simulink model "bldcm_model"  (R2023b)
settings: Solver=ode23s  StartTime=0.0  StopTime=10  RelTol=1e-3
libraries: spsMosfetLib x6, eeGeneralControl x3, simulink x1, spsDCVoltageSourceLib x1, spsGroundLib x1, slpidlib x1, spsThreePhaseSeriesRLCBranchLib x1, spsThreePhaseVIMeasurementLib x1, sps_lib x1
settings Model: Creator=nicog  LastModifiedBy=nicog

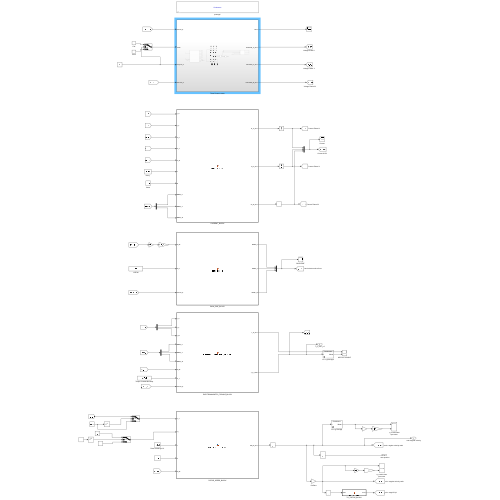
[thumbnail: Simulink's stored preview of the top-level diagram]
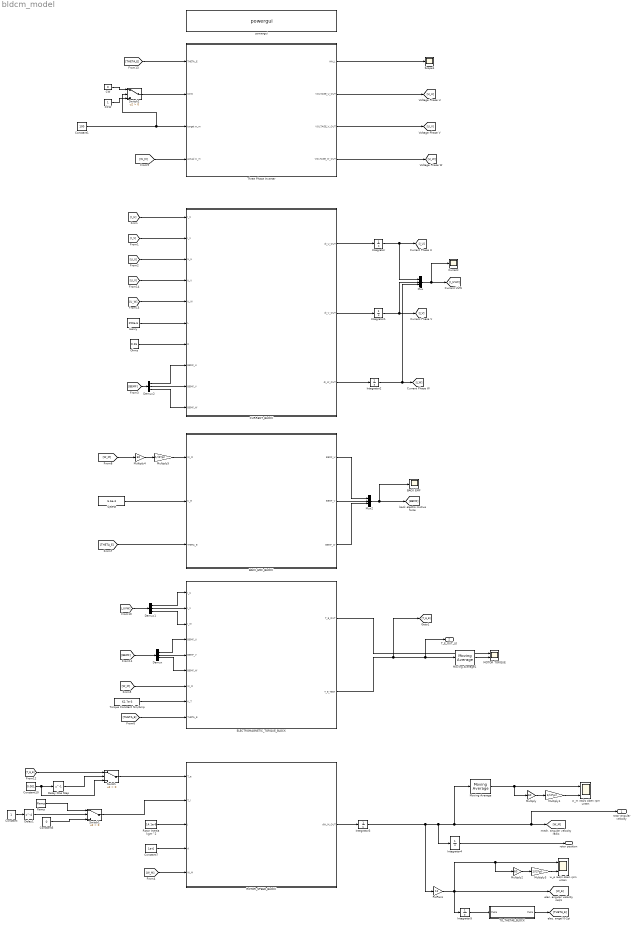
== system bldcm_model ==
  BACK EMF : Scope
  BACK_EMF_BLOCK : MATLAB Function  TreatAsAtomicUnit=on
  CCW : Constant
  CURRENT_BLOCK : MATLAB Function  TreatAsAtomicUnit=on
  CW : Constant  Value=0
  Constant : Constant
  Constant1 : Constant  Value=100
  Constant10 : Constant  Value=0.001
  Constant5 : Constant  Value=0
  Constant7 : Constant  Value=1e-6
  Current : Scope
  Delay One Step : Delay  DelayLength=1
  Delay1 : Delay  DelayLength=4
  Demux : Demux  Outputs=3
  Demux1 : Demux  Outputs=3
  Demux2 : Demux  Outputs=3
  ELECTROMAGNETIC_TORQUE_BLOCK : MATLAB Function  TreatAsAtomicUnit=on
  Henry : Constant  Value=250e-6
  Integrator{,1..5} (6 alike) : Integrator
  MOTOR TORQUE : Scope  NumInputPorts=2
  Moving Average : eeGeneralControl/Moving Average  VariantControl=Variant1  LabelModeActiveChoice=Continuous  f=30  x0=0  BufferSize=8192  Ts=0
      settings: LibrarySourceBlock=ee_sl_lib/General Control/Moving Average
  Moving Average1 : eeGeneralControl/Moving Average  VariantControl=Variant1  LabelModeActiveChoice=Continuous  f=30  x0=0  BufferSize=8192  Ts=0
      settings: LibrarySourceBlock=ee_sl_lib/General Control/Moving Average
  Multiply : Gain  Gain=60
  Multiply1 : Gain  Gain=1/(2*pi)
  Multiply2 : Gain  Gain=60
  Multiply3 : Gain  Gain=1/(2*pi)
  Multiply4 : Gain  Gain=60
  Multiply5 : Gain  Gain=1/(2*pi)
  Mux : Mux  Inputs=3
  Mux2 : Mux  Inputs=3
  Ohms : Constant  Value=0.26
  PolPairs : Gain  Gain=12
  ROTOR_SPEED_BLOCK : MATLAB Function  TreatAsAtomicUnit=on
  Ramp : simulink/Sources/Ramp  slope=1  start=1  InitialOutput=1
  Rotor Inertia kgm^2 : Constant  Value=14.1e-6
  Scope1 : Scope
  Switch : Switch  Criteria=u2 > Threshold  SaturateOnIntegerOverflow=off  InputSameDT=off
  Switch1 : Switch  Criteria=u2 > Threshold  SaturateOnIntegerOverflow=off  InputSameDT=off
  Switch2 : Switch  Criteria=u2 > Threshold  SaturateOnIntegerOverflow=off  InputSameDT=off
  TO_THETAE_BLOCK : MATLAB Function  TreatAsAtomicUnit=on
  Three Phase Inverter : Subsystem
  Torque Constant Nm/Amp : Constant  Value=62.7e-3
  V/RPM : Constant  Value=6.6e-3
  powergui : sps_lib/powergui  Priority=1  SimulationMode=Continuous  SampleTime=50e-6  frequency=60  Iterations=50  frequencyindice=0  Pbase=100e6  ErrMax=1e-4  UnitsV=kV  UnitsW=MW  buscounter=0  FunctionMessages=off  echomessages=off  EnableUseOfTLC=off  CurrentSourceSwitches=off  DisableSnubberDevices=off  DisableRonSwitches=off  DisableVfSwitches=off  DisplayEquations=off  AutomaticDiscreteSolvers=off  SolverType=Tustin/Backward Euler (TBE)  Interpol=off  ExternalGateDelay=off  methode=off  Ts=100  x0status=blocks  SPID=on  SwTol=0  HookPort=off  NonlinearTolerance=1e-4  nMaxIteration=100  ContinueOnMaxIteration=off  RestoreLinks=warning  ResistiveCurrentMeasurement=off  Frange=[0:2:500]  Ylog=off  Xlog=on  ShowGrid=off  save=off  variable=ZData  structure=0  ZoomFFT=off  StartTime=0.0  cycles=1  DisplayStyle=1  fundamental=60  FreqAxis=off  MaxFrequency=1000  frequencyindicesteady=1  RmsSteady=1  display=off
  w_e rad/s oben rpm unten : Scope  NumInputPorts=2
  w_m rad/s oben rpm unten : Scope  NumInputPorts=2
  rotor angular velocity : Outport
  T_E_OUT_L0 : Outport  Port=2
  rotor position : Outport  Port=3
  wires:
  PolPairs/1 -> [W_E], Multiply2/1, w_e rad/s oben rpm unten/1, Integrator5/1
  TO_THETAE_BLOCK/1(theta) -> [THETA_E]
  Integrator5/1 -> TO_THETAE_BLOCK/1("theta ")
  Constant1/1 -> Switch2/2, Three Phase Inverter/3(target w_m)
  CCW/1 -> Switch2/3
  Constant5/1 -> Switch1/3
  BACK_EMF_BLOCK/2(BEMF_V) -> Mux2/2
  Ramp/1 -> Switch1/1
  Moving Average1/1 -> MOTOR TORQUE/2
  Integrator4/1 -> rotor position/1
  Three Phase Inverter/4(VOLTAGE_W_OUT) -> [U_W]
  Rotor Inertia kgm^2/1 -> ROTOR_SPEED_BLOCK/3(J)
  [W_M] -> ROTOR_SPEED_BLOCK/5(W_M)
  Demux1/2 -> ELECTROMAGNETIC_TORQUE_BLOCK/2(I_V)
  Demux1/1 -> ELECTROMAGNETIC_TORQUE_BLOCK/1(I_U)
  Multiply/1 -> Multiply1/1
  Integrator1/1 -> [I_V], Mux/2
  ROTOR_SPEED_BLOCK/1(dW_M_OUT) -> Integrator3/1
  Demux/3 -> ELECTROMAGNETIC_TORQUE_BLOCK/6(BEMF_W)
  Delay One Step/1 -> Switch/2
  CURRENT_BLOCK/2(dI_V_OUT) -> Integrator1/1
  Moving Average/1 -> Multiply/1, w_m rad/s oben rpm unten/1
  CURRENT_BLOCK/1(dI_U_OUT) -> Integrator/1
  ELECTROMAGNETIC_TORQUE_BLOCK/1(T_E_OUT) -> MOTOR TORQUE/1
  [BEMF] -> Demux2/1
  ELECTROMAGNETIC_TORQUE_BLOCK/2(T_E_TEST) -> T_E_OUT_L0/1, Moving Average1/1, [T_E_B]
  Demux2/3 -> CURRENT_BLOCK/10(BEMF_W)
  [U_U] -> CURRENT_BLOCK/3(U_U)
  Torque Constant Nm/Amp/1 -> ELECTROMAGNETIC_TORQUE_BLOCK/8(K_T)
  Integrator2/1 -> [I_W], Mux/3
  Constant/1 -> Delay1/1
  [I_V] -> CURRENT_BLOCK/2(I_V)
  [THETA_E] -> ELECTROMAGNETIC_TORQUE_BLOCK/9(THETA_E)
  [W_M] -> Multiply4/1
  Demux2/1 -> CURRENT_BLOCK/8(BEMF_U)
  Constant10/1 -> Delay One Step/1, Switch/3
  Multiply2/1 -> Multiply3/1
  [U_W] -> CURRENT_BLOCK/5(U_W)
  [I_UVW] -> Demux1/1
  Integrator3/1 -> PolPairs/1, Integrator4/1, Moving Average/1, rotor angular velocity/1, [W_M]
  Multiply3/1 -> w_e rad/s oben rpm unten/2
  Integrator/1 -> [I_U], Mux/1
  Demux1/3 -> ELECTROMAGNETIC_TORQUE_BLOCK/3(I_W)
  Switch2/1 -> Three Phase Inverter/2(CCW)
  Constant7/1 -> ROTOR_SPEED_BLOCK/4(d)
  Demux/1 -> ELECTROMAGNETIC_TORQUE_BLOCK/4(BEMF_U)
  Demux2/2 -> CURRENT_BLOCK/9(BEMF_V)
  V/RPM/1 -> BACK_EMF_BLOCK/2(K_E)
  Multiply1/1 -> w_m rad/s oben rpm unten/2
  Delay1/1 -> Switch1/2
  [I_U] -> CURRENT_BLOCK/1(I_U)
  BACK_EMF_BLOCK/3(BEMF_W) -> Mux2/3
  Multiply5/1 -> BACK_EMF_BLOCK/1(W_M)
  Switch/1 -> ROTOR_SPEED_BLOCK/1(T_e)
  [W_M] -> ELECTROMAGNETIC_TORQUE_BLOCK/7(W_M)
  [BEMF] -> Demux/1
  Henry/1 -> CURRENT_BLOCK/6(L)
  CW/1 -> Switch2/1
  Three Phase Inverter/3(VOLTAGE_V_OUT) -> [U_V]
  BACK_EMF_BLOCK/1(BEMF_U) -> Mux2/1
  [U_V] -> CURRENT_BLOCK/4(U_V)
  [T_E_B] -> Switch/1
  Three Phase Inverter/2(VOLTAGE_U_OUT) -> [U_U]
  Mux/1 -> Current/1, [I_UVW]
  Ohms/1 -> CURRENT_BLOCK/7(R)
  [W_M] -> Three Phase Inverter/4(actual w_m)
  Three Phase Inverter/1(HALL) -> Scope1/1
  Multiply4/1 -> Multiply5/1
  Mux2/1 -> BACK EMF/1, [BEMF]
  CURRENT_BLOCK/3(dI_W_OUT) -> Integrator2/1
  Demux/2 -> ELECTROMAGNETIC_TORQUE_BLOCK/5(BEMF_V)
  [THETA_E] -> BACK_EMF_BLOCK/3(THETA_E)
  [THETA_E] -> Three Phase Inverter/1(THETA_E)
  Switch1/1 -> ROTOR_SPEED_BLOCK/2(T_l)

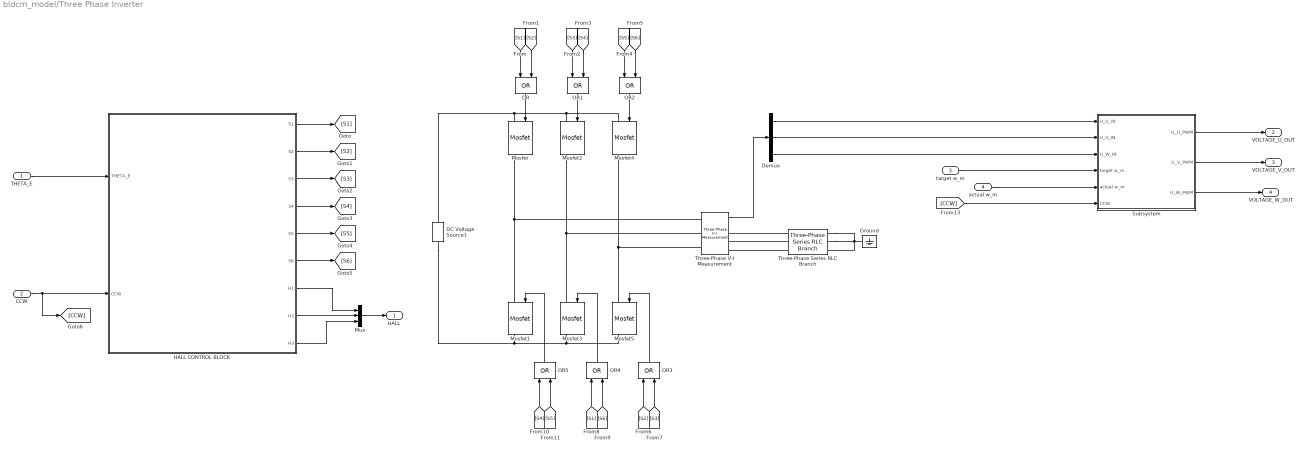
== system bldcm_model/Three Phase Inverter ==
  THETA_E : Inport
  CCW : Inport  Port=2
  target w_m : Inport  Port=3
  actual w_m : Inport  Port=4
  DC Voltage Source1 : spsDCVoltageSourceLib/DC Voltage Source  Amplitude=48  Measurements=None
  Demux : Demux  Outputs=3
  Ground : spsGroundLib/Ground  LConnTagsString=a
  HALL CONTROL BLOCK : MATLAB Function  TreatAsAtomicUnit=on
  Mosfet{,1..5} (6 alike) : spsMosfetLib/Mosfet  Ron=0.1  Lon=0  Rd=0.01  Vfd=0  IC=0  Rs=1e5  Cs=inf  Measurements=on
  Mux : Mux  Inputs=3
  OR{,1..5} (6 alike) : Logic  Operator=OR  IconShape=distinctive  AllPortsSameDT=off  OutDataTypeStr=boolean
  Subsystem : Subsystem
  Three-Phase Series RLC Branch : spsThreePhaseSeriesRLCBranchLib/Three-Phase Series RLC Branch  LConnTagsString=A|B|C  RConnTagsString=A|B|C  BranchType=RL  Resistance=100000  Inductance=0.3e-3  Capacitance=1e-6  Measurements=None
  Three-Phase V-I Measurement : spsThreePhaseVIMeasurementLib/Three-Phase V-I Measurement  VoltageMeasurement=phase-to-ground  SetLabelV=off  LabelV=Vabc  Vpu=off  VpuLL=off  CurrentMeasurement=yes  SetLabelI=off  LabelI=Iabc  Ipu=off  Pbase=100e6  Vbase=500e3  OutputType=Complex  PhasorSimulation=off  PSBequivalent=0
  HALL : Outport
  VOLTAGE_U_OUT : Outport  Port=2
  VOLTAGE_V_OUT : Outport  Port=3
  VOLTAGE_W_OUT : Outport  Port=4
  wires:
  Three-Phase V-I Measurement/1 -> Demux/1
  Demux/1 -> Subsystem/1(U_U_IN)
  Demux/2 -> Subsystem/2(U_V_IN)
  Demux/3 -> Subsystem/3(U_W_IN)
  OR/1 -> Mosfet/1
  HALL CONTROL BLOCK/1(S1) -> [S1]
  [S1] -> OR/1
  HALL CONTROL BLOCK/2(S2) -> [S2]
  [S2] -> OR/2
  [S4] -> OR1/2
  [S3] -> OR1/1
  OR1/1 -> Mosfet2/1
  [S6] -> OR2/2
  [S5] -> OR2/1
  OR2/1 -> Mosfet4/1
  HALL CONTROL BLOCK/4(S4) -> [S4]
  HALL CONTROL BLOCK/3(S3) -> [S3]
  HALL CONTROL BLOCK/5(S5) -> [S5]
  HALL CONTROL BLOCK/6(S6) -> [S6]
  [S3] -> OR3/2
  [S4] -> OR5/1
  [S5] -> OR5/2
  [S6] -> OR4/2
  [S2] -> OR3/1
  [S1] -> OR4/1
  OR5/1 -> Mosfet1/1
  OR4/1 -> Mosfet3/1
  OR3/1 -> Mosfet5/1
  THETA_E/1 -> HALL CONTROL BLOCK/1(THETA_E)
  HALL CONTROL BLOCK/7(H1) -> Mux/1
  HALL CONTROL BLOCK/8(H2) -> Mux/2
  HALL CONTROL BLOCK/9(H3) -> Mux/3
  Mux/1 -> HALL/1
  Subsystem/1(U_U_PWM) -> VOLTAGE_U_OUT/1
  Subsystem/3(U_W_PWM) -> VOLTAGE_W_OUT/1
  Subsystem/2(U_V_PWM) -> VOLTAGE_V_OUT/1
  CCW/1 -> [CCW], HALL CONTROL BLOCK/2(CCW)
  [CCW] -> Subsystem/6(CCW)
  target w_m/1 -> Subsystem/4(target w_m)
  actual w_m/1 -> Subsystem/5(actual w_m)
  connections:
  Three-Phase V-I Measurement/LConn3 -- Mosfet5/LConn1 -- Mosfet4/RConn1
  Mosfet1/RConn1 -- DC Voltage Source1/LConn1 -- Mosfet5/RConn1 -- Mosfet3/RConn1
  Mosfet/LConn1 -- DC Voltage Source1/RConn1 -- Mosfet4/LConn1 -- Mosfet2/LConn1
  Mosfet1/LConn1 -- Mosfet/RConn1 -- Three-Phase V-I Measurement/LConn1
  Three-Phase V-I Measurement/LConn2 -- Mosfet3/LConn1 -- Mosfet2/RConn1
  Three-Phase Series RLC Branch/RConn3 -- Three-Phase Series RLC Branch/RConn2 -- Ground/LConn1 -- Three-Phase Series RLC Branch/RConn1
  Three-Phase Series RLC Branch/LConn1 -- Three-Phase V-I Measurement/RConn1
  Three-Phase Series RLC Branch/LConn2 -- Three-Phase V-I Measurement/RConn2
  Three-Phase Series RLC Branch/LConn3 -- Three-Phase V-I Measurement/RConn3

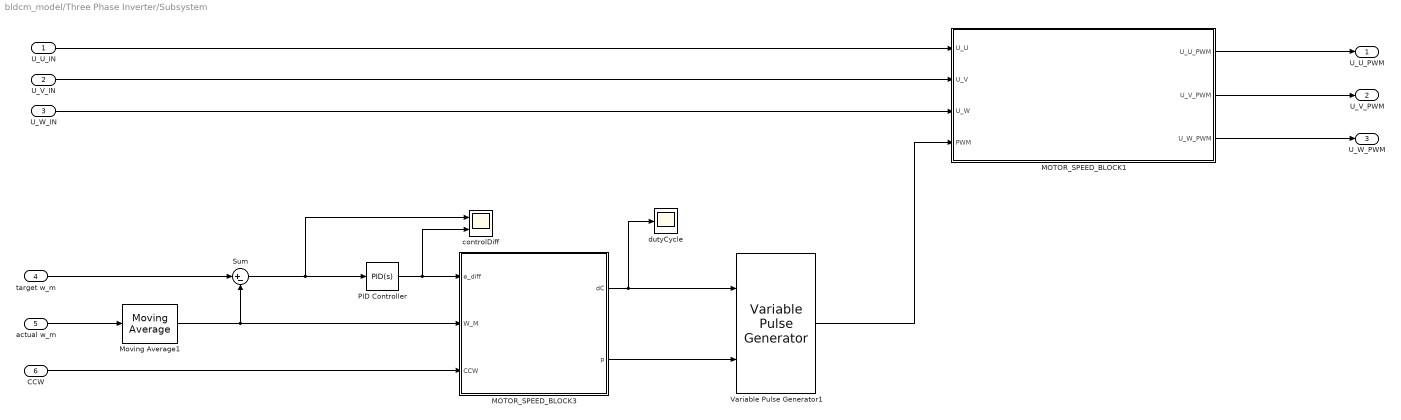
== system bldcm_model/Three Phase Inverter/Subsystem ==
  U_U_IN : Inport
  U_V_IN : Inport  Port=2
  U_W_IN : Inport  Port=3
  target w_m : Inport  Port=4
  actual w_m : Inport  Port=5
  CCW : Inport  Port=6
  MOTOR_SPEED_BLOCK1 : MATLAB Function  TreatAsAtomicUnit=on
  MOTOR_SPEED_BLOCK3 : MATLAB Function  TreatAsAtomicUnit=on
  Moving Average1 : eeGeneralControl/Moving Average  VariantControl=Variant1  LabelModeActiveChoice=Continuous  f=60  x0=0  BufferSize=8192  Ts=0
      settings: LibrarySourceBlock=ee_sl_lib/General Control/Moving Average
  PID Controller : slpidlib/PID Controller  Controller=PID  Form=Parallel  TimeDomain=Continuous-time  UseExternalTs=off  SampleTime=-1  IntegratorMethod=Forward Euler  FilterMethod=Forward Euler  ControllerParametersSource=internal  P=0.2  I=1  UseKiTs=off  D=0  N=100  UseFilter=on  TunerSelectOption=Transfer Function Based (PID Tuner App)  InitialConditionSource=internal  InitialConditionForIntegrator=0  InitialConditionForFilter=0  DifferentiatorICPrevScaledInput=0  ExternalReset=none  TrackingMode=off  Kt=1  LimitOutput=off  SatLimitsSource=internal  UpperSaturationLimit=inf  LowerSaturationLimit=-inf  LinearizeAsGain=on  AntiWindupMode=none  Kb=1  LimitIntegrator=off  UpperIntegratorSaturationLimit=inf  LowerIntegratorSaturationLimit=-inf  POutMin=[]  POutMax=[]  IOutMin=[]  IOutMax=[]  DOutMin=[]  DOutMax=[]  NOutMin=[]  NOutMax=[]  SumOutMin=[]  SumOutMax=[]  SaturationOutMin=[]  SaturationOutMax=[]  PParamMin=[]  PParamMax=[]  IParamMin=[]  IParamMax=[]  DParamMin=[]  DParamMax=[]  NParamMin=[]  NParamMax=[]  KbParamMin=[]  KbParamMax=[]  KtParamMin=[]  KtParamMax=[]  KbOutMin=[]  KbOutMax=[]  KtOutMin=[]  KtOutMax=[]  IntegratorOutMin=[]  IntegratorOutMax=[]  FilterOutMin=[]  FilterOutMax=[]  SumI1OutMin=[]  SumI1OutMax=[]  SumI2OutMin=[]  SumI2OutMax=[]  SumI3OutMin=[]  SumI3OutMax=[]  SumI4OutMin=[]  SumI4OutMax=[]  SumDOutMin=[]  SumDOutMax=[]  DifferentiatorOutMin=[]  DifferentiatorOutMax=[]  FilterDiffOutCoefMin=[]  FilterDiffOutCoefMax=[]  ReciprocalOutMin=[]  ReciprocalOutMax=[]  SumDenOutMin=[]  SumDenOutMax=[]  SumNumOutMin=[]  SumNumOutMax=[]  DivideOutMin=[]  DivideOutMax=[]  UdiffTsProdOutMin=[]  UdiffTsProdOutMax=[]  NTsProdOutMin=[]  NTsProdOutMax=[]  UintegralTsProdOutMin=[]  UintegralTsProdOutMax=[]  UngainTsProdOutMin=[]  UngainTsProdOutMax=[]  ClampingZeroOutDataTypeStr=Inherit: Inherit via back propagation  ClampingZeroOutMin=[]  ClampingZeroOutMax=[]  FilterDenConstantOutDataTypeStr=Inherit: Inherit via back propagation  FilterDenConstantOutMin=[]  FilterDenConstantOutMax=[]  PCopyOutDataTypeStr=Inherit: Inherit via back propagation  PCopyOutMin=[]  PCopyOutMax=[]  NCopyOutDataTypeStr=Inherit: Inherit via back propagation  NCopyOutMin=[]  NCopyOutMax=[]  IntegratorContinuousStateAttributes=''  IntegratorStateMustResolveToSignalObject=off  IntegratorRTWStateStorageClass=Auto  FilterContinuousStateAttributes=''  FilterStateMustResolveToSignalObject=off  FilterRTWStateStorageClass=Auto  ParallelPVariant=InternalParameters  IdealPVariant=Disabled  IVariant=InternalParameters  DVariant=InternalParameters  IntegratorVariant=Continuous  SatVariant=Disabled  AWVariant=Passthrough  PCopyVariant=Disabled  TRVariant=Disabled  FdbkBlocksVariant=Forward  IdealPFdbkVariant=Disabled  SatFdbkVariant=Disabled  DerivativeFilterVariant=ContFilter  NVariant=InternalParameters  NCopyVariant=Disabled  FilterICVariant=InternalICsFilter  IntegratorICVariant=InternalICs  ExternalResetVariant=Disabled  TRSumVariant=Passthrough  SumFdbkVariant=Disabled  SumVariant=Sum_PID  TsampFilterVariant=InternalTs  TsampNgainVariant=Passthrough  TsampIntegralVariant=Disabled_SignalSpec  ExternalSaturationOutDataTypeStr=Inherit: Same as second input
  Sum : Sum  Inputs=|+-
  Variable Pulse Generator1 : VariablePulseGenerator  AllowZeroPulseWidth=on  SampleTime=0.1
  controlDiff : Scope  NumInputPorts=2
  dutyCycle : Scope
  U_U_PWM : Outport
  U_V_PWM : Outport  Port=2
  U_W_PWM : Outport  Port=3
  wires:
  target w_m/1 -> Sum/1
  CCW/1 -> MOTOR_SPEED_BLOCK3/3(CCW)
  MOTOR_SPEED_BLOCK3/1(dC) -> Variable Pulse Generator1/1, dutyCycle/1
  MOTOR_SPEED_BLOCK3/2(p) -> Variable Pulse Generator1/2
  Variable Pulse Generator1/1 -> MOTOR_SPEED_BLOCK1/4(PWM)
  U_U_IN/1 -> MOTOR_SPEED_BLOCK1/1(U_U)
  U_V_IN/1 -> MOTOR_SPEED_BLOCK1/2(U_V)
  U_W_IN/1 -> MOTOR_SPEED_BLOCK1/3(U_W)
  MOTOR_SPEED_BLOCK1/1(U_U_PWM) -> U_U_PWM/1
  MOTOR_SPEED_BLOCK1/2(U_V_PWM) -> U_V_PWM/1
  MOTOR_SPEED_BLOCK1/3(U_W_PWM) -> U_W_PWM/1
  Sum/1 -> PID Controller/1, controlDiff/1
  actual w_m/1 -> Moving Average1/1
  Moving Average1/1 -> MOTOR_SPEED_BLOCK3/2(W_M), Sum/2
  PID Controller/1 -> controlDiff/2, MOTOR_SPEED_BLOCK3/1(e_diff)

== matlab function bldcm_model/Three Phase Inverter/HALL CONTROL BLOCK ==
  data: S1 output; S2 output; S3 output; S4 output; S5 output; S6 output; THETA_E input; H1 output; H2 output; H3 output; CCW input
function [S1, S2, S3, S4, S5, S6, H1, H2 ,H3] = HALL_BLOCK(THETA_E, CCW)
%#codegen

% Normalisierung
%THETA_E = mod(THETA_E, 2*pi);
% Initialisieren Sie alle Signale auf 0

THETA = mod(THETA_E,  2*pi);

% electrical theta 0°-60°
if (0 <= THETA) && (THETA < 1*pi/3)
    H1 = 1;
    H2 = 0;
    H3 = 1;

% electrical theta 60°-120°
elseif (1*pi/3 <= THETA) &&(THETA < 2*pi/3)
    H1 = 1;
    H2 = 0;
    H3 = 0;
% electrical theta 120°-180°
elseif (2*pi/3 <= THETA) && (THETA < pi)
    H1 = 1;
    H2 = 1;
    H3 = 0;

% electrical theta 180°-240°
elseif (pi <= THETA) && (THETA < 4*pi/3)
    H1 = 0;
    H2 = 1;
    H3 = 0;

% electrical theta 240°-300°
elseif (4*pi/3 <= THETA) && (THETA < 5*pi/3)
    H1 = 0;
    H2 = 1;
    H3 = 1;

% electrical theta 300°-360°
elseif (5*pi/3 <= THETA) && (THETA < 2*pi)
    H1 = 0;
    H2 = 0;
    H3 = 1;

% something went wrong
else
    H1 = 0;
    H2 = 0;
    H3 = 0;
end

if CCW ~= 1
    if (H1 == 1) && (H3 == 1)
       S3 = 0; S2 = 0; S4 = 0; S5 = 0; S6 = 0;
       S1 = 1;
    elseif (H1 == 1) && (H2 ~= 1 && H3 ~= 1)
       S1 = 0; S4 = 0; S3 = 0; S5 = 0; S6 = 0;
       S2 = 1;
    elseif (H1 == 1) && (H2 == 1)
       S1 = 0; S2 = 0; S5 = 0; S4 = 0; S6 = 0;
       S3 = 1;
    elseif (H2 == 1) && (H1 ~= 1 && H3 ~= 1)
       S1 = 0; S2 = 0; S3 = 0; S6 = 0; S5 = 0;
       S4 = 1;
    elseif (H2 == 1) && (H3 == 1)
       S2 = 0; S3 = 0; S4 = 0; S1 = 0; S6 = 0;
       S5 = 1;
    elseif (H3 == 1) && (H1 ~= 1 && H2 ~= 1)
       S1 = 0; S3 = 0; S4 = 0; S5 = 0; S2 = 0;
       S6 = 1;
    else
       S1 = 0; S2 = 0; S3 = 0; S4 = 0; S5 = 0; S6 = 0; 
    end
else
    if (H1 == 1) && (H3 == 1)
       S3 = 0; S2 = 0; S1 = 0; S5 = 0; S6 = 0;
       S4 = 1;
    elseif (H1 == 1) && (H2 ~= 1 && H3 ~= 1)
       S1 = 0; S4 = 0; S3 = 0; S2 = 0; S6 = 0;
       S5 = 1;
    elseif (H1 == 1) && (H2 == 1)
       S1 = 0; S2 = 0; S5 = 0; S4 = 0; S3 = 0;
       S6 = 1;
    elseif (H2 == 1) && (H1 ~= 1 && H3 ~= 1)
       S4 = 0; S2 = 0; S3 = 0; S6 = 0; S5 = 0;
       S1 = 1;
    elseif (H2 == 1) && (H3 == 1)
       S5 = 0; S3 = 0; S4 = 0; S1 = 0; S6 = 0;
       S2 = 1;
    elseif (H3 == 1) && (H1 ~= 1 && H2 ~= 1)
       S1 = 0; S6 = 0; S4 = 0; S5 = 0; S2 = 0;
       S3 = 1;
    else
       S1 = 0; S2 = 0; S3 = 0; S4 = 0; S5 = 0; S6 = 0; 
    end
end

end

== matlab function bldcm_model/Three Phase Inverter/Subsystem/MOTOR_SPEED_BLOCK1 ==
  data: U_U input; U_V input; U_W input; U_U_PWM output; PWM input; U_V_PWM output; U_W_PWM output
function [U_U_PWM, U_V_PWM, U_W_PWM] = PWM_SPEED_BLOCK(U_U, U_V, U_W, PWM)
%#codegen

%    This function was generated by the Symbolic Math Toolbox version 23.2.
%    20-Mar-2024 19:58:52

U_U_PWM = 0;
U_V_PWM = 0;
U_W_PWM = 0;

% Apply PWM scaling based on input and PWM signal
if U_U ~= 0 && PWM ~= 0
    U_U_PWM = U_U * PWM;
end
if U_V ~= 0 && PWM ~= 0
    U_V_PWM = U_V * PWM;
end
if U_W ~= 0 && PWM ~= 0
    U_W_PWM = U_W * PWM;
end

end

== matlab function bldcm_model/Three Phase Inverter/Subsystem/MOTOR_SPEED_BLOCK3 ==
  data: e_diff input; dC output; W_M input; CCW input; p output
function [dC, p] = PWM_SPEED_BLOCK(e_diff, W_M, CCW)
%#codegen

%    This function was generated by the Symbolic Math Toolbox version 23.2.
%    20-Mar-2024 19:58:52

%I = Ki * integral;
%D = Kd * derivative;

if CCW == 1
    e_diff = e_diff * (-1);
end

if W_M == 0
    p = 0.001;
elseif W_M < 0
    p = 1/(W_M*(-20));
else
    p = 1/(W_M*20);
end

p = max(1e-4, min(0.001, p));

% Sigmoidfunktion
dC = 1/(1+exp(-e_diff));
dC = max(0, min(0.99, dC));

end

== matlab function bldcm_model/BACK_EMF_BLOCK ==
  data: W_M input; K_E input; THETA_E input; BEMF_U output; BEMF_V output; BEMF_W output
function [BEMF_U, BEMF_V, BEMF_W] = BEMF_BLOCK(W_M, K_E, THETA_E)
%#codegen

%    This function was generated by the Symbolic Math Toolbox version 23.2.
%    20-Mar-2024 19:08:31

%THETA = mod(THETA_E,  2*pi);
THETA = THETA_E;
% electrical theta 0°-60°
if (0 <= THETA) && (THETA < 1*pi/3)
    F_U = 1;
    F_V = -1;
    F_W = 1-6*THETA/pi;

% electrical theta 60°-120°
elseif (1*pi/3 <= THETA) &&(THETA < 2*pi/3)
    F_U = 1;
    F_V = 6*THETA/pi - 3;
    F_W = -1;

% electrical theta 120°-180°
elseif (2*pi/3 <= THETA) && (THETA < pi)
    F_U = -6*THETA/pi + 5;
    F_V = 1;
    F_W = -1;

% electrical theta 180°-240°
elseif (pi <= THETA) && (THETA < 4*pi/3)
    F_U = -1;
    F_V = 1;
    F_W = 6*THETA/pi -7;

% electrical theta 240°-300°
elseif (4*pi/3 <= THETA) && (THETA < 5*pi/3)
    F_U = -1;
    F_V = -6*THETA/pi + 9;
    F_W = 1;

% electrical theta 300°-360°
elseif (5*pi/3 <= THETA) && (THETA < 2*pi)
    F_U = 6*THETA/pi - 11;
    F_V = -1;
    F_W = 1;

% something went wrong
else
    F_U = NaN;
    F_V = NaN;
    F_W = NaN;
end

BEMF_U = K_E*W_M*F_U;
BEMF_V = K_E*W_M*F_V;
BEMF_W = K_E*W_M*F_W;

end

== matlab function bldcm_model/CURRENT_BLOCK ==
  data: I_U input; dI_U_OUT output; I_V input; U_U input; U_V input; U_W input; L input; R input; BEMF_U input; BEMF_V input; BEMF_W input; dI_V_OUT output; dI_W_OUT output
function [dI_U_OUT,dI_V_OUT,dI_W_OUT] = CURRENT_BLOCK(I_U,I_V,U_U,U_V,U_W,L,R,BEMF_U,BEMF_V,BEMF_W)
%#codegen

%    This function was generated by the Symbolic Math Toolbox version 23.2.
%    20-Mar-2024 19:08:31

% https://de.mathworks.com/matlabcentral/answers/446003-relation-between-flux-linkage-and-voltage-constant-power_pmsynchronousmachineparams
% based on the link the magnetic flux is approximately lamda
%LAMDA = (sqrt(2)/sqrt(3)) * ((48/sqrt(2))/P*W_M)
%LAMDA = 1/sqrt(3) * (K_T/1000*P) * (60/2*pi)

%U_UV = U_U - U_V;
%U_VW = U_V - U_W;

%dI_U_OUT = (U_UV.*2.0+U_VW-I_U.*R.*3.0+P*MFLUX*W_M*(-EMF_U.*2.0+EMF_V+EMF_W))./(L.*3.0);

%dI_V_OUT = (-U_UV+U_VW-I_V.*R.*3.0+P*MFLUX*W_M*(EMF_U-EMF_V.*2.0+EMF_W))./(L.*3.0);

%dI_W_OUT = -(dI_U_OUT+dI_V_OUT);

E_UW = BEMF_U - BEMF_W;
E_WV = BEMF_W - BEMF_V;

U_UW = U_U - U_W;
U_WV = U_W - U_V;

dI_U_OUT = (U_UW.*2.0 + U_WV - I_U.*R.*3.0 - E_UW.*2.0 - E_WV)./(L.*3.0);
dI_V_OUT = (-U_UW - U_WV.*2.0 - I_V.*R.*3.0 + E_UW + E_WV.*2.0)./(L.*3.0);
dI_W_OUT = -(dI_U_OUT+dI_V_OUT);

%dI_U_OUT = -(R*I_U)/L - (P*W_M*EMF_U)/(2*L) + U_U/L
%dI_V_OUT = -(R*I_V)/L - (P*W_M*EMF_V)/(2*L) + U_V/L
%dI_W_OUT = -(R*I_W)/L - (P*W_M*EMF_W)/(2*L) + U_W/L
%dI_W_OUT = -(dI_U_OUT+dI_V_OUT)
end

== matlab function bldcm_model/ELECTROMAGNETIC_TORQUE_BLOCK ==
  data: I_U input; I_V input; I_W input; BEMF_U input; BEMF_V input; BEMF_W input; W_M input; T_E_OUT output; K_T input; THETA_E input; T_E_TEST output
function [T_E_OUT,T_E_TEST] = ELECTROMAGNETIC_TORQUE_BLOCK(I_U, I_V, I_W, BEMF_U, BEMF_V, BEMF_W, W_M, K_T, THETA_E)
%#codegen

%    This function was generated by the Symbolic Math Toolbox version 23.2.
%    20-Mar-2024 15:56:32

T_E_OUT = ((BEMF_U*I_U+BEMF_V*I_V+BEMF_W*I_W)./W_M);

%THETA = mod(THETA_E,  2*pi);
THETA = THETA_E;
% electrical theta 0°-60°
if (0 <= THETA) && (THETA < 1*pi/3)
    F_U = 1;
    F_V = -1;
    F_W = 1-6*THETA/pi;

% electrical theta 60°-120°
elseif (1*pi/3 <= THETA) &&(THETA < 2*pi/3)
    F_U = 1;
    F_V = 6*THETA/pi - 3;
    F_W = -1;

% electrical theta 120°-180°
elseif (2*pi/3 <= THETA) && (THETA < pi)
    F_U = -6*THETA/pi + 5;
    F_V = 1;
    F_W = -1;

% electrical theta 180°-240°
elseif (pi <= THETA) && (THETA < 4*pi/3)
    F_U = -1;
    F_V = 1;
    F_W = 6*THETA/pi -7;

% electrical theta 240°-300°
elseif (4*pi/3 <= THETA) && (THETA < 5*pi/3)
    F_U = -1;
    F_V = -6*THETA/pi + 9;
    F_W = 1;

% electrical theta 300°-360°
elseif (5*pi/3 <= THETA) && (THETA < 2*pi)
    F_U = 6*THETA/pi - 11;
    F_V = -1;
    F_W = 1;

% something went wrong
else
    F_U = NaN;
    F_V = NaN;
    F_W = NaN;
end

T_E_TEST = K_T*((F_U*I_U)+(F_V*I_V)+(F_W*I_W));

end

== matlab function bldcm_model/ROTOR_SPEED_BLOCK ==
  data: T_e input; T_l input; J input; d input; dW_M_OUT output; W_M input
function dW_M_OUT = MOTOR_SPEED_BLOCK(T_e,T_l,J,d,W_M)
%#codegen

%    This function was generated by the Symbolic Math Toolbox version 23.2.
%    20-Mar-2024 19:58:52

dW_M_OUT = -(-T_e+T_l+W_M.*d)./J;
end

== matlab function bldcm_model/TO_THETAE_BLOCK ==
  data: theta output; theta input
function theta = generateTheta(theta)
    theta = mod(theta, 2*pi);
end
